simulink model "missile2"  (R2023b)
settings: Solver=ode4  StartTime=0.0  StopTime=40  FixedStep=0.001  RelTol=1e-3
settings Model: Creator=Tanish  LastModifiedBy=Tanish
settings OptimizationCC: DefaultParameterBehavior=Inlined  EnhancedBackFolding=on  PassReuseOutputArgsAs=Individual arguments  ZeroExternalMemoryAtStartup=off  ZeroInternalMemoryAtStartup=off  OptimizeBlockOrder=speed  DifferentSizesBufferReuse=on  OptimizationCustomize=off  EfficientTunableParamExpr=on
settings DebuggingCC: ParameterTunabilityLossMsg=error
settings SFSimCC: MATLABDynamicMemAlloc=off
settings RTWCC: Description=Embedded Coder  SystemTargetFile=ert.tlc  TemplateMakefile=ert_default_tmf
settings CodeAppCC: ForceParamTrailComments=on  IgnoreCustomStorageClasses=off  OperatorAnnotations=on  SimulinkDataObjDesc=on  SFDataObjDesc=on  InsertBlockDesc=on
settings ERTTargetCC: TargetLangStandard=C99 (ISO)  GenerateSampleERTMain=on  InlinedParameterPlacement=NonHierarchical  ERTCustomFileTemplate=example_file_process.tlc

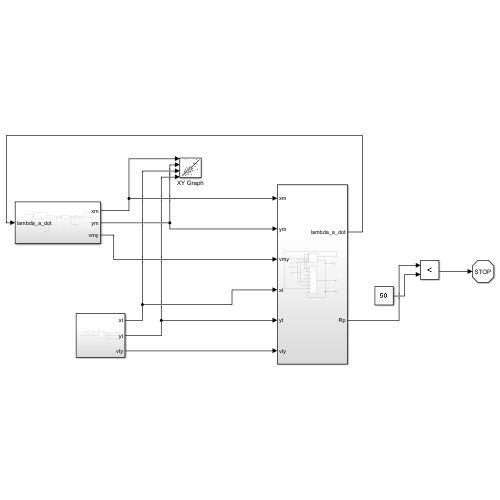
[thumbnail: Simulink's stored preview of the top-level diagram]
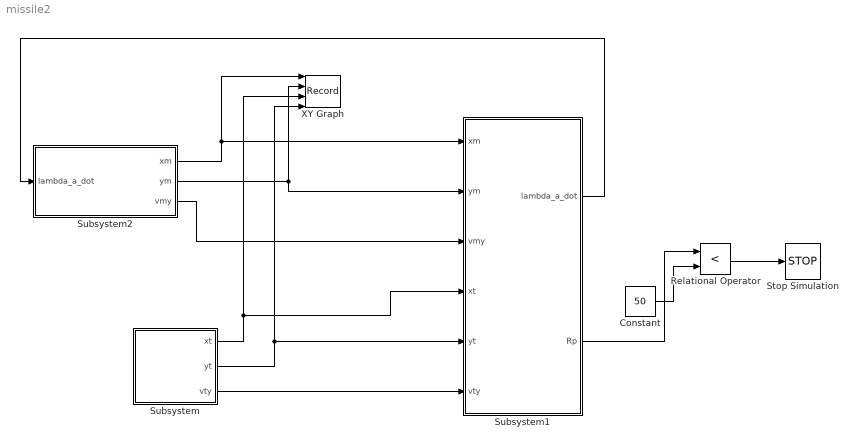
== system missile2 ==
  Constant : Constant  Value=50
  Relational Operator : RelationalOperator  Operator=<  OutDataTypeStr=boolean  RndMeth=Simplest  InputSameDT=off
  Stop Simulation : Stop
  Subsystem : Subsystem
  Subsystem1 : Subsystem
  Subsystem2 : Subsystem
  XY Graph : Record  FileSettingsInternal="{\"entries\":[{\"content\":{\"excelSettings\":{\"content\":{},\"type\":\"Streamout.ExcelSettings\"}},\"type\":\"Streamout.FileSettingStorage\",\"uuid\":\"\"}],\"packageUris\":[\"http:\\/\\/schema.mathworks.com\\/mf0\\/streamout_blocks\\/R2020a\"],\"version\":\"1.0\"}"  Layout=[1 1]  SignalsInternal="{\"entries\":[{\"content\":{\"signals\":[{\"content\":{\"blockPath\":[],\"dimensions\":[1],\"domain\":\"\",\"lineColor\":\"#a2142f\",\"plots\":[1],\"port\":1,\"signalID\":8,\"signalName\":\"Subsystem2:1\"},\"type\":\"RecordBlkView.Signal\",\"uuid\":\"\"},{\"content\":{\"blockPath\":[],\"dimensions\":[1],\"domain\":\"\",\"lineColor\":\"#139fff\",\"plots\":[1],\"port\":2,\"signalID\":11,\"signalName\":\"Subsystem2:2\"},\"type\":\"RecordBlkView.Signal\",\"uuid\":\"\"},{\"content\":{\"blockPath\":[],\"dimensions\":[1],\"domain\":\"\",\"lineColor\":\"#0072bd\",\"plots\":[1],\"port\":3,\"signalID\":14,\"signalName\":\"Subsystem:1\"},\"type\":\"RecordBlkView.Signal\",\"uuid\":\"\"},{\"content\":{\"blockPath\":[],\"dimensions\":[1],\"domain\":\"\",\"lineColor\":\"#d95319\",\"plots\":[1],\"port\":4,\"signalID\":17,\"signalName\":\"Subsystem:2\"},\"type\":\"RecordBlkView.Signal\",\"uuid\":\"\"}]},\"type\":\"RecordBlkView.InputSignals\",\"uuid\":\"\"}],\"packageUris\":[\"http:\\/\\/schema.mathworks.com\\/mf0\\/streamout_blocks\\/R2020a\"],\"version\":\"1.0\"}"  VisualizationBindings="{\"xyplotplugin\":{\"info\":[{\"series\":[{\"bindingParametersList\":[{\"parameter\":\"X-Axis\",\"signalID\":8,\"signalName\":\"Subsystem2:1\"},{\"parameter\":\"Y-Axis\",\"signalID\":11,\"signalName\":\"Subsystem2:2\"}],\"seriesID\":44510},{\"bindingParametersList\":[{\"parameter\":\"X-Axis\",\"signalID\":14,\"signalName\":\"Subsystem:1\"},{\"parameter\":\"Y-Axis\",\"signalID\":17,\"signalName\":\"Subsystem:2\"}],\"seriesID\":1600}],\"subplotID\":1}]}}"  CompatibilityTag=XY
  wires:
  Subsystem/1(xt) -> XY Graph/3, Subsystem1/4(xt)
  Subsystem1/1(lambda_a_dot) -> Subsystem2/1(lambda_a_dot)
  Subsystem2/1(xm) -> XY Graph/1, Subsystem1/1(xm)
  Subsystem2/2(ym) -> XY Graph/2, Subsystem1/2(ym)
  Relational Operator/1 -> Stop Simulation/1
  Constant/1 -> Relational Operator/2
  Subsystem1/2(Rp) -> Relational Operator/1
  Subsystem2/3(vmy) -> Subsystem1/3(vmy)
  Subsystem/3(vty) -> Subsystem1/6(vty)
  Subsystem/2(yt) -> XY Graph/4, Subsystem1/5(yt)

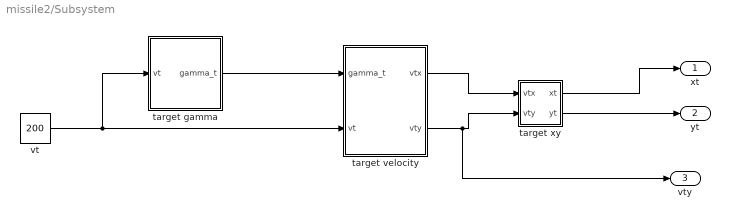
== system missile2/Subsystem ==
  target gamma : Subsystem
  target velocity : Subsystem
  target xy : Subsystem
  vt : Constant  Value=200
  xt : Outport
  yt : Outport  Port=2
  vty : Outport  Port=3
  wires:
  vt/1 -> target gamma/1(vt), target velocity/2(vt)
  target xy/2(yt) -> yt/1
  target velocity/1(vtx) -> target xy/1(vtx)
  target gamma/1(gamma_t) -> target velocity/1(gamma_t)
  target velocity/2(vty) -> vty/1, target xy/2(vty)
  target xy/1(xt) -> xt/1

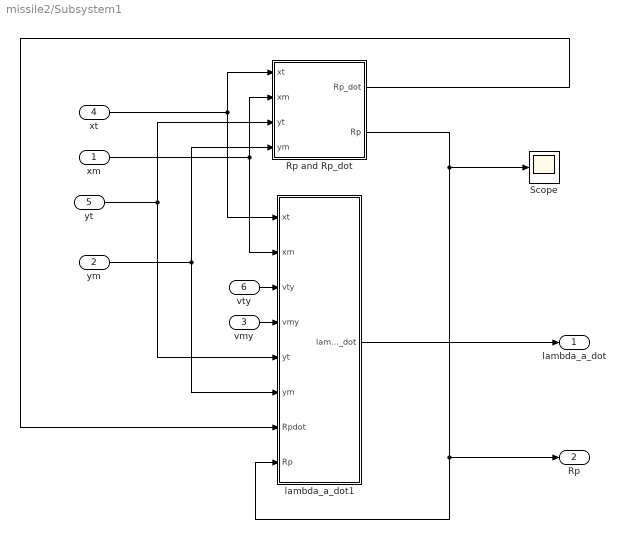
== system missile2/Subsystem1 ==
  xm : Inport
  ym : Inport  Port=2
  vmy : Inport  Port=3
  xt : Inport  Port=4
  yt : Inport  Port=5
  vty : Inport  Port=6
  Rp and Rp_dot : Subsystem
  Scope : Scope
  lambda_a_dot1 : Subsystem
  lambda_a_dot : Outport
  Rp : Outport  Port=2
  wires:
  vty/1 -> lambda_a_dot1/3(vty)
  lambda_a_dot1/1(lambda_a_dot) -> lambda_a_dot/1
  vmy/1 -> lambda_a_dot1/4(vmy)
  xm/1 -> lambda_a_dot1/2(xm), Rp and Rp_dot/2(xm)
  Rp and Rp_dot/1(Rp_dot) -> lambda_a_dot1/7(Rpdot)
  ym/1 -> lambda_a_dot1/6(ym), Rp and Rp_dot/4(ym)
  xt/1 -> Rp and Rp_dot/1(xt), lambda_a_dot1/1(xt)
  yt/1 -> Rp and Rp_dot/3(yt), lambda_a_dot1/5(yt)
  Rp and Rp_dot/2(Rp) -> Scope/1, Rp/1, lambda_a_dot1/8(Rp)

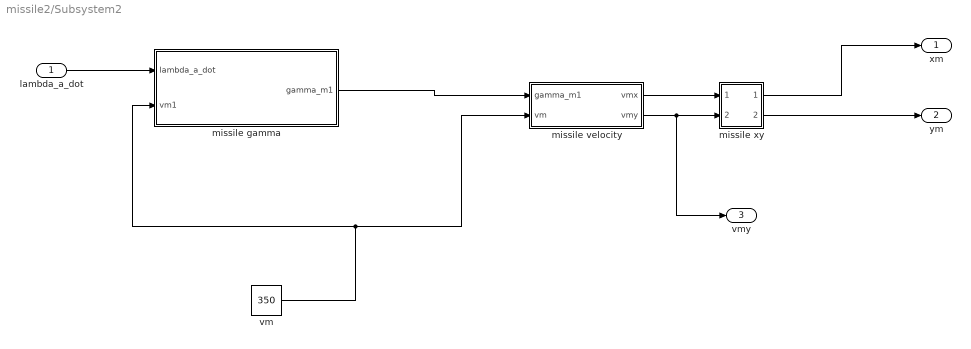
== system missile2/Subsystem2 ==
  lambda_a_dot : Inport
  missile gamma : Subsystem
  missile velocity : Subsystem
  missile xy : Subsystem
  vm : Constant  Value=350
  xm : Outport
  ym : Outport  Port=2
  vmy : Outport  Port=3
  wires:
  missile xy/1(xm) -> xm/1
  missile gamma/1(gamma_m1) -> missile velocity/1(gamma_m1)
  vm/1 -> missile gamma/2(vm1), missile velocity/2(vm)
  lambda_a_dot/1 -> missile gamma/1(lambda_a_dot)
  missile xy/2(ym) -> ym/1
  missile velocity/1(vmx) -> missile xy/1(vmx)
  missile velocity/2(vmy) -> vmy/1, missile xy/2(vmy)

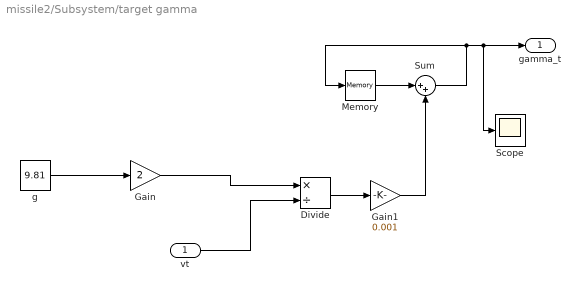
== system missile2/Subsystem/target gamma ==
  vt : Inport
  Divide : Product  Inputs=*/
  Gain : Gain  Gain=2
  Gain1 : Gain  Gain=0.001
  Memory : Memory  InitialCondition=(-170*pi)/180  InheritSampleTime=on  LinearizeAsDelay=on
  Scope : Scope
  Sum : Sum  Inputs=|++
  g : Constant  Value=9.81
  gamma_t : Outport
  wires:
  Gain/1 -> Divide/1
  vt/1 -> Divide/2
  Gain1/1 -> Sum/2
  Sum/1 -> Scope/1, gamma_t/1, Memory/1
  Memory/1 -> Sum/1
  g/1 -> Gain/1
  Divide/1 -> Gain1/1

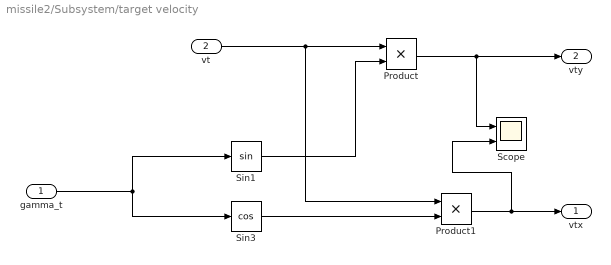
== system missile2/Subsystem/target velocity ==
  gamma_t : Inport
  vt : Inport  Port=2
  Product : Product
  Product1 : Product
  Scope : Scope  NumInputPorts=2
  Sin1 : Trigonometry
  Sin3 : Trigonometry  Operator=cos
  vtx : Outport
  vty : Outport  Port=2
  wires:
  Sin3/1 -> Product1/2
  gamma_t/1 -> Sin1/1, Sin3/1
  Sin1/1 -> Product/2
  Product/1 -> Scope/1, vty/1
  vt/1 -> Product1/1, Product/1
  Product1/1 -> Scope/2, vtx/1

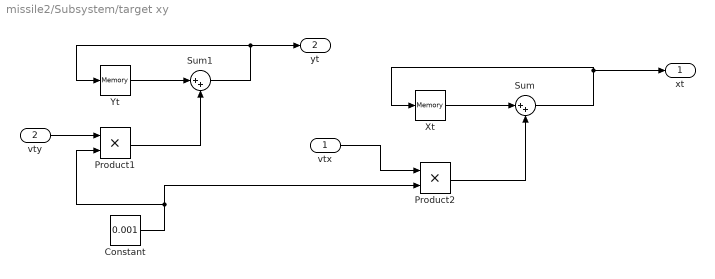
== system missile2/Subsystem/target xy ==
  vtx : Inport
  vty : Inport  Port=2
  Constant : Constant  Value=0.001
  Product1 : Product
  Product2 : Product
  Sum : Sum  Inputs=|++
  Sum1 : Sum  Inputs=|++
  Xt : Memory  InitialCondition=10000  InheritSampleTime=on  LinearizeAsDelay=on
  Yt : Memory  InitialCondition=500  InheritSampleTime=on  LinearizeAsDelay=on
  xt : Outport
  yt : Outport  Port=2
  wires:
  Sum/1 -> xt/1, Xt/1
  Product1/1 -> Sum1/2
  Yt/1 -> Sum1/1
  Constant/1 -> Product2/2, Product1/2
  Xt/1 -> Sum/1
  Product2/1 -> Sum/2
  vtx/1 -> Product2/1
  Sum1/1 -> yt/1, Yt/1
  vty/1 -> Product1/1

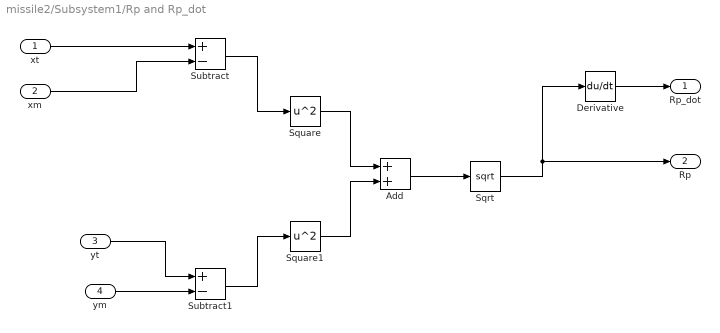
== system missile2/Subsystem1/Rp and Rp_dot ==
  xt : Inport
  xm : Inport  Port=2
  yt : Inport  Port=3
  ym : Inport  Port=4
  Add : Sum
  Derivative : Derivative
  Sqrt : Sqrt
  Square : Math  Operator=square
  Square1 : Math  Operator=square
  Subtract : Sum  Inputs=+-
  Subtract1 : Sum  Inputs=+-
  Rp_dot : Outport
  Rp : Outport  Port=2
  wires:
  Sqrt/1 -> Rp/1, Derivative/1
  Derivative/1 -> Rp_dot/1
  Add/1 -> Sqrt/1
  Square1/1 -> Add/2
  Square/1 -> Add/1
  Subtract1/1 -> Square1/1
  Subtract/1 -> Square/1
  ym/1 -> Subtract1/2
  yt/1 -> Subtract1/1
  xm/1 -> Subtract/2
  xt/1 -> Subtract/1

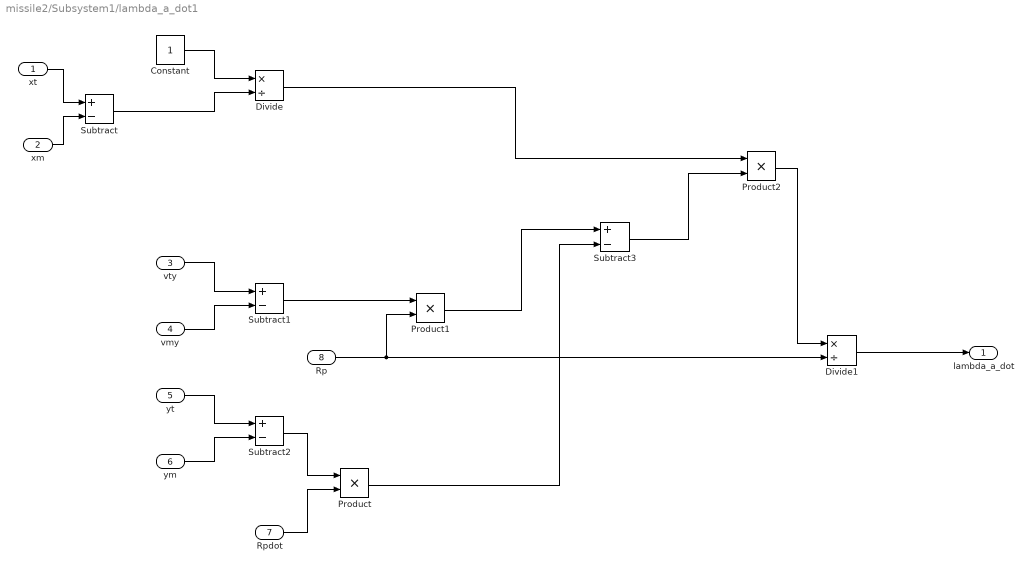
== system missile2/Subsystem1/lambda_a_dot1 ==
  xt : Inport
  xm : Inport  Port=2
  vty : Inport  Port=3
  vmy : Inport  Port=4
  yt : Inport  Port=5
  ym : Inport  Port=6
  Rpdot : Inport  Port=7
  Rp : Inport  Port=8
  Constant : Constant
  Divide : Product  Inputs=*/
  Divide1 : Product  Inputs=*/
  Product : Product
  Product1 : Product
  Product2 : Product
  Subtract{,1..3} (4 alike) : Sum  Inputs=+-
  lambda_a_dot : Outport
  wires:
  xt/1 -> Subtract/1
  xm/1 -> Subtract/2
  vty/1 -> Subtract1/1
  vmy/1 -> Subtract1/2
  yt/1 -> Subtract2/1
  ym/1 -> Subtract2/2
  Subtract2/1 -> Product/1
  Rpdot/1 -> Product/2
  Subtract1/1 -> Product1/1
  Constant/1 -> Divide/1
  Subtract/1 -> Divide/2
  Product1/1 -> Subtract3/1
  Product/1 -> Subtract3/2
  Divide/1 -> Product2/1
  Subtract3/1 -> Product2/2
  Rp/1 -> Divide1/2, Product1/2
  Product2/1 -> Divide1/1
  Divide1/1 -> lambda_a_dot/1

== system missile2/Subsystem2/missile gamma ==
  lambda_a_dot : Inport
  vm1 : Inport  Port=2
  gamma_m : Subsystem
  gamma_m_dot : Subsystem
  gamma_m1 : Outport
  wires:
  vm1/1 -> gamma_m_dot/2(vm1)
  gamma_m_dot/1(gamma_m_dot) -> gamma_m/1(gamma_m_dot)
  gamma_m/1(gamma_m) -> gamma_m1/1
  lambda_a_dot/1 -> gamma_m_dot/1(lambda_a_dot)

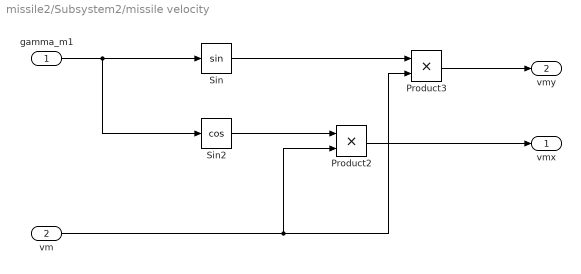
== system missile2/Subsystem2/missile velocity ==
  gamma_m1 : Inport
  vm : Inport  Port=2
  Product2 : Product
  Product3 : Product
  Sin : Trigonometry
  Sin2 : Trigonometry  Operator=cos
  vmx : Outport
  vmy : Outport  Port=2
  wires:
  Product3/1 -> vmy/1
  Sin2/1 -> Product2/1
  vm/1 -> Product3/2, Product2/2
  Product2/1 -> vmx/1
  gamma_m1/1 -> Sin2/1, Sin/1
  Sin/1 -> Product3/1

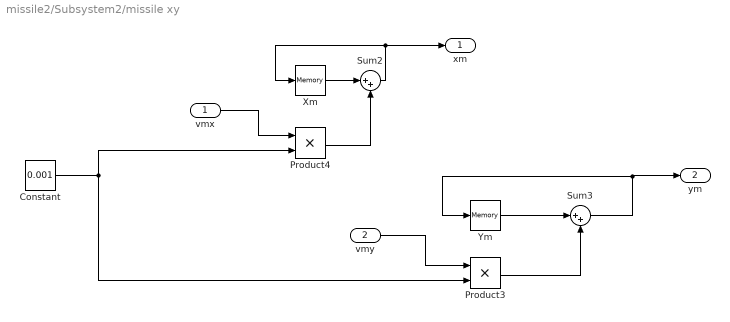
== system missile2/Subsystem2/missile xy ==
  vmx : Inport
  vmy : Inport  Port=2
  Constant : Constant  Value=0.001
  Product3 : Product
  Product4 : Product
  Sum2 : Sum  Inputs=|++
  Sum3 : Sum  Inputs=|++
  Xm : Memory  InheritSampleTime=on  LinearizeAsDelay=on
  Ym : Memory  InheritSampleTime=on  LinearizeAsDelay=on
  xm : Outport
  ym : Outport  Port=2
  wires:
  Ym/1 -> Sum3/1
  Product4/1 -> Sum2/2
  vmy/1 -> Product3/1
  Constant/1 -> Product4/2, Product3/2
  Product3/1 -> Sum3/2
  Sum2/1 -> xm/1, Xm/1
  Sum3/1 -> ym/1, Ym/1
  vmx/1 -> Product4/1
  Xm/1 -> Sum2/1

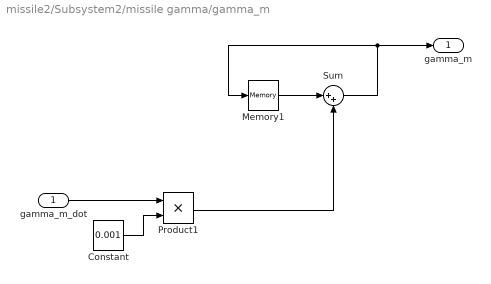
== system missile2/Subsystem2/missile gamma/gamma_m ==
  gamma_m_dot : Inport
  Constant : Constant  Value=0.001
  Memory1 : Memory  InitialCondition=pi/18  InheritSampleTime=on  LinearizeAsDelay=on
  Product1 : Product
  Sum : Sum  Inputs=|++
  gamma_m : Outport
  wires:
  Constant/1 -> Product1/2
  Sum/1 -> gamma_m/1, Memory1/1
  Memory1/1 -> Sum/1
  Product1/1 -> Sum/2
  gamma_m_dot/1 -> Product1/1

== system missile2/Subsystem2/missile gamma/gamma_m_dot ==
  lambda_a_dot : Inport
  vm1 : Inport  Port=2
  Divide : Product  Inputs=*/
  N_yaw : Constant  Value=3
  Product : Product  Inputs=3
  gamma_m_dot : Outport
  wires:
  lambda_a_dot/1 -> Product/2
  vm1/1 -> Divide/2, Product/3
  Product/1 -> Divide/1
  N_yaw/1 -> Product/1
  Divide/1 -> gamma_m_dot/1
